simulink model "Pendulum6DOF"  (R2017a)
settings: Solver=ode45  StartTime=0.0  StopTime=500  MaxStep=0.01  RelTol=1e-3
settings Model: Creator=Charlie  LastModifiedBy=Charlie

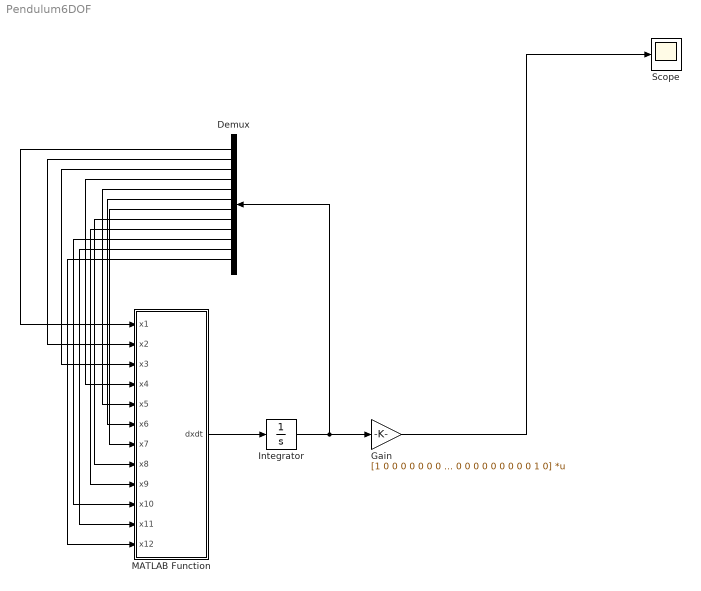
== system Pendulum6DOF ==
  Demux : Demux  Outputs=12
  Gain : Gain  Gain=[1 0 0 0 0 0 0 0 0 0 0 0; 0 0 1 0 0 0 0 0 0 0 0 0; 0 0 0 0 1 0 0 0 0 0 0 0; 0 0 0 0 0 0 1 0 0 0 0 0; 0 0 0 0 0 0 0 0 1 0 0 0; 0 0 0 0 0 0 0 0 0 0 1 0]  Multiplication=Matrix(K*u)
  Integrator : Integrator  InitialCondition=[pi-1;0;pi-0.2;0; 0;0; 1.5;0; 6;0; 0;0]
  MATLAB Function : MATLAB Function  TreatAsAtomicUnit=on
  Scope : Scope
  wires:
  Integrator/1 -> Demux/1, Gain/1
  Gain/1 -> Scope/1
  Demux/6 -> MATLAB Function/6(x6)
  Demux/5 -> MATLAB Function/5(x5)
  Demux/4 -> MATLAB Function/4(x4)
  Demux/3 -> MATLAB Function/3(x3)
  Demux/2 -> MATLAB Function/2(x2)
  Demux/1 -> MATLAB Function/1(x1)
  Demux/7 -> MATLAB Function/7(x7)
  Demux/8 -> MATLAB Function/8(x8)
  Demux/9 -> MATLAB Function/9(x9)
  Demux/10 -> MATLAB Function/10(x10)
  Demux/11 -> MATLAB Function/11(x11)
  Demux/12 -> MATLAB Function/12(x12)
  MATLAB Function/1(dxdt) -> Integrator/1

== matlab function Pendulum6DOF/MATLAB Function ==
  data: x1 input; dxdt output; x2 input; x3 input; x4 input; x5 input; x6 input; x7 input; x8 input; x9 input; x10 input; x11 input; x12 input
%function dxdt = dynamics(K,x)
function dxdt = dynamics(x1,x2,x3,x4,x5,x6,x7,x8,x9,x10,x11,x12)

dxdt = [x2;
    -((10430973*cos(x3)*sin(x1))/250000000 + (1029*x4^2*sin(2*x1))/5000000 + (50421*x4^2*cos(x1)^3*sin(x1))/50000 + (7066143*cos(x1)^2*cos(x3)*sin(x1))/250000 - (53851*x2*x4*sin(2*x3))/50000000 - (7066143*cos(x1)^2*cos(x3)^3*sin(x1))/250000000 + (10633*x2^2*cos(x1)*cos(x3)^2*sin(x1))/50000000 + (53851*x4^2*cos(x1)*cos(x3)^2*sin(x1))/50000000 - (31899*x6^2*cos(x1)*cos(x3)^2*sin(x1))/25000000 + (1029*x4*x6*cos(x1)^2*cos(x3))/1250000 + (50421*x4*x6*cos(x1)^4*cos(x3))/25000 + (7203*x2^2*cos(x1)^3*cos(x3)^2*sin(x1))/50000 - (7203*x2^2*cos(x1)^3*cos(x3)^4*sin(x1))/50000000 - (21609*x4^2*cos(x1)^3*cos(x3)^2*sin(x1))/25000000 - (7203*x4^2*cos(x1)^3*cos(x3)^4*sin(x1))/50000000 - (21609*x6^2*cos(x1)^3*cos(x3)^2*sin(x1))/25000 + (21609*x6^2*cos(x1)^3*cos(x3)^4*sin(x1))/25000000 + (21609*x4*x6*cos(x1)^2*cos(x3)^3)/12500000 - (3623109*x4*x6*cos(x1)^4*cos(x3)^3)/12500000 + (53851*x2*x4*cos(x1)^2*cos(x3)*sin(x3))/25000000 + (7203*x2*x4*cos(x1)^2*cos(x3)^3*sin(x3))/25000000 - (7203*x2*x4*cos(x1)^4*cos(x3)^3*sin(x3))/25000000 - (21609*x2*x6*cos(x1)*cos(x3)^2*sin(x1)*sin(x3))/12500000 + (7203*x2*x6*cos(x1)^3*cos(x3)^2*sin(x1)*sin(x3))/25000)/((50495431*cos(x1)^2)/50000000 + (53851*cos(x3)^2)/50000000 - (5386129*cos(x1)^2*cos(x3)^2)/2500000000 - (7203*cos(x1)^2*cos(x3)^4)/50000000 - (7210203*cos(x1)^4*cos(x3)^2)/50000000 + (7203*cos(x1)^4*cos(x3)^4)/25000000 + 1030519/2500000000);
    x4;
    ((50495431*x2*x4*sin(2*x1))/50000000 - (7076573973*cos(x1)*sin(x3))/250000000 + (7066143*cos(x1)^3*cos(x3)^2*sin(x3))/250000000 - (7213633*x2^2*cos(x1)^2*cos(x3)*sin(x3))/50000000 - (53851*x4^2*cos(x1)^2*cos(x3)*sin(x3))/50000000 - (3579891*x4^2*cos(x1)^4*cos(x3)*sin(x3))/25000000 + (21640899*x6^2*cos(x1)^2*cos(x3)*sin(x3))/25000000 + (21640899*x2*x6*cos(x1)^2*cos(x3))/12500000 + (7203*x2^2*cos(x1)^4*cos(x3)^3*sin(x3))/50000000 + (7203*x4^2*cos(x1)^4*cos(x3)^3*sin(x3))/50000000 - (21609*x6^2*cos(x1)^4*cos(x3)^3*sin(x3))/25000000 + (3579891*x2*x6*cos(x1)^2*cos(x3)^3)/12500000 - (7203*x2*x6*cos(x1)^4*cos(x3)^3)/25000 - (53851*x2*x4*cos(x1)*cos(x3)^2*sin(x1))/25000000 - (7210203*x2*x4*cos(x1)^3*cos(x3)^2*sin(x1))/25000000 + (7203*x2*x4*cos(x1)^3*cos(x3)^4*sin(x1))/25000000 + (3579891*x4*x6*cos(x1)^3*cos(x3)^2*sin(x1)*sin(x3))/12500000)/((50495431*cos(x1)^2)/50000000 + (53851*cos(x3)^2)/50000000 - (5386129*cos(x1)^2*cos(x3)^2)/2500000000 - (7203*cos(x1)^2*cos(x3)^4)/50000000 - (7210203*cos(x1)^4*cos(x3)^2)/50000000 + (7203*cos(x1)^4*cos(x3)^4)/25000000 + 1030519/2500000000);
    x6;
    -(147*((17157*x2*x4*cos(x3))/25000000 - (48069*cos(x3)*sin(x1)*sin(x3))/5000000 + (343*x4^2*cos(x1)^3*sin(x1)*sin(x3))/1000000 + (48069*cos(x1)^2*cos(x3)*sin(x1)*sin(x3))/5000000 - (17157*x2*x4*cos(x1)^2*cos(x3))/25000000 - (49*x2*x4*cos(x1)^2*cos(x3)^3)/500000 + (49*x2*x4*cos(x1)^4*cos(x3)^3)/500000 + (7*x4^2*cos(x1)*sin(x1)*sin(x3))/50000000 - (49*x2^2*cos(x1)*cos(x3)^2*sin(x1)*sin(x3))/1000000 + (147*x6^2*cos(x1)*cos(x3)^2*sin(x1)*sin(x3))/500000 + (14707*x2*x6*cos(x1)*cos(x3)^2*sin(x1))/25000000 + (49*x2*x6*cos(x1)*cos(x3)^4*sin(x1))/500000 + (7*x4*x6*cos(x1)^2*cos(x3)*sin(x3))/25000000 + (343*x4*x6*cos(x1)^4*cos(x3)*sin(x3))/500000 + (49*x2^2*cos(x1)^3*cos(x3)^2*sin(x1)*sin(x3))/1000000 - (49*x4^2*cos(x1)^3*cos(x3)^2*sin(x1)*sin(x3))/1000000 - (147*x6^2*cos(x1)^3*cos(x3)^2*sin(x1)*sin(x3))/500000 + (49*x2*x6*cos(x1)^3*cos(x3)^2*sin(x1))/500000 - (49*x2*x6*cos(x1)^3*cos(x3)^4*sin(x1))/250000 + (49*x4*x6*cos(x1)^2*cos(x3)^3*sin(x3))/500000 - (49*x4*x6*cos(x1)^4*cos(x3)^3*sin(x3))/250000))/(50*((50495431*cos(x1)^2)/50000000 + (53851*cos(x3)^2)/50000000 - (5386129*cos(x1)^2*cos(x3)^2)/2500000000 - (7203*cos(x1)^2*cos(x3)^4)/50000000 - (7210203*cos(x1)^4*cos(x3)^2)/50000000 + (7203*cos(x1)^4*cos(x3)^4)/25000000 + 1030519/2500000000));
    x8;
    ((1030519*x7*x12^2)/2500000000 - (1030519*x10*x12)/1250000000 - (50495431*x10*x12*cos(x1)^2)/25000000 - (53851*x10*x12*cos(x3)^2)/25000000 + (50495431*x7*x12^2*cos(x1)^2)/50000000 + (53851*x7*x12^2*cos(x3)^2)/50000000 - (5386129*x7*x12^2*cos(x1)^2*cos(x3)^2)/2500000000 - (7203*x7*x12^2*cos(x1)^2*cos(x3)^4)/50000000 - (7210203*x7*x12^2*cos(x1)^4*cos(x3)^2)/50000000 + (7203*x7*x12^2*cos(x1)^4*cos(x3)^4)/25000000 + (5386129*x10*x12*cos(x1)^2*cos(x3)^2)/1250000000 + (7203*x10*x12*cos(x1)^2*cos(x3)^4)/25000000 + (7210203*x10*x12*cos(x1)^4*cos(x3)^2)/25000000 - (7203*x10*x12*cos(x1)^4*cos(x3)^4)/12500000 - (336483*cos(x3)*cos(x5)*cos(x11)*sin(x3))/500000000 + (1030519*x2^2*cos(x5)*sin(x1)*sin(x11))/50000000000 - (1030519*x2^2*cos(x11)*sin(x1)*sin(x5))/50000000000 + (1030519*x6^2*cos(x5)*sin(x1)*sin(x11))/50000000000 - (1030519*x6^2*cos(x11)*sin(x1)*sin(x5))/50000000000 - (336483*cos(x3)*sin(x3)*sin(x5)*sin(x11))/500000000 + (1030519*x2*x6*cos(x1)*sin(x5)*sin(x11))/25000000000 + (50495431*x2^2*cos(x1)^3*cos(x5)*cos(x11)*sin(x3))/1000000000 + (2230529*x4^2*cos(x1)^3*cos(x5)*cos(x11)*sin(x3))/50000000000 + (50471421*x4^2*cos(x1)^5*cos(x5)*cos(x11)*sin(x3))/1000000000 + (50495431*x6^2*cos(x1)^3*cos(x5)*cos(x11)*sin(x3))/1000000000 + (336483*cos(x1)^2*cos(x3)*cos(x5)*cos(x11)*sin(x3))/250000000 + (7073209143*cos(x1)^4*cos(x3)*cos(x5)*cos(x11)*sin(x3))/5000000000 + (50495431*x2^2*cos(x1)^2*cos(x5)*sin(x1)*sin(x11))/1000000000 - (50495431*x2^2*cos(x1)^2*cos(x11)*sin(x1)*sin(x5))/1000000000 + (53851*x2^2*cos(x3)^2*cos(x5)*sin(x1)*sin(x11))/1000000000 - (53851*x2^2*cos(x3)^2*cos(x11)*sin(x1)*sin(x5))/1000000000 + (1030029*x4^2*cos(x1)^2*cos(x5)*sin(x1)*sin(x11))/50000000000 - (1030029*x4^2*cos(x1)^2*cos(x11)*sin(x1)*sin(x5))/50000000000 + (50471421*x4^2*cos(x1)^4*cos(x5)*sin(x1)*sin(x11))/1000000000 - (50471421*x4^2*cos(x1)^4*cos(x11)*sin(x1)*sin(x5))/1000000000 + (50495431*x6^2*cos(x1)^2*cos(x5)*sin(x1)*sin(x11))/1000000000 - (50495431*x6^2*cos(x1)^2*cos(x11)*sin(x1)*sin(x5))/1000000000 + (53851*x6^2*cos(x3)^2*cos(x5)*sin(x1)*sin(x11))/1000000000 - (53851*x6^2*cos(x3)^2*cos(x11)*sin(x1)*sin(x5))/1000000000 + (7066143*cos(x1)*cos(x3)^3*cos(x5)*sin(x1)*sin(x11))/5000000000 - (7066143*cos(x1)*cos(x3)^3*cos(x11)*sin(x1)*sin(x5))/5000000000 + (7073209143*cos(x1)^3*cos(x3)*cos(x5)*sin(x1)*sin(x11))/5000000000 - (7073209143*cos(x1)^3*cos(x3)*cos(x11)*sin(x1)*sin(x5))/5000000000 + (50495431*x2^2*cos(x1)^3*sin(x3)*sin(x5)*sin(x11))/1000000000 + (2230529*x4^2*cos(x1)^3*sin(x3)*sin(x5)*sin(x11))/50000000000 + (50471421*x4^2*cos(x1)^5*sin(x3)*sin(x5)*sin(x11))/1000000000 + (50495431*x6^2*cos(x1)^3*sin(x3)*sin(x5)*sin(x11))/1000000000 + (336483*cos(x1)^2*cos(x3)*sin(x3)*sin(x5)*sin(x11))/250000000 + (7073209143*cos(x1)^4*cos(x3)*sin(x3)*sin(x5)*sin(x11))/5000000000 + (50495431*x2*x6*cos(x1)^3*cos(x5)*cos(x11))/500000000 + (50495431*x2*x6*cos(x1)^3*sin(x5)*sin(x11))/500000000 + (7066143*cos(x1)^2*cos(x3)^3*cos(x5)*cos(x11)*sin(x3))/5000000000 - (7066143*cos(x1)^4*cos(x3)^3*cos(x5)*cos(x11)*sin(x3))/2500000000 - (7066143*cos(x1)^3*cos(x3)^3*cos(x5)*sin(x1)*sin(x11))/2500000000 + (7066143*cos(x1)^3*cos(x3)^3*cos(x11)*sin(x1)*sin(x5))/2500000000 + (7066143*cos(x1)^2*cos(x3)^3*sin(x3)*sin(x5)*sin(x11))/5000000000 - (7066143*cos(x1)^4*cos(x3)^3*sin(x3)*sin(x5)*sin(x11))/2500000000 + (1030519*x2^2*cos(x1)*cos(x5)*cos(x11)*sin(x3))/50000000000 + (49*x4^2*cos(x1)*cos(x5)*cos(x11)*sin(x3))/5000000000 + (1030519*x6^2*cos(x1)*cos(x5)*cos(x11)*sin(x3))/50000000000 + (336483*cos(x1)*cos(x3)*cos(x5)*sin(x1)*sin(x11))/500000000 - (336483*cos(x1)*cos(x3)*cos(x11)*sin(x1)*sin(x5))/500000000 + (1030519*x2^2*cos(x1)*sin(x3)*sin(x5)*sin(x11))/50000000000 + (49*x4^2*cos(x1)*sin(x3)*sin(x5)*sin(x11))/5000000000 + (1030519*x6^2*cos(x1)*sin(x3)*sin(x5)*sin(x11))/50000000000 + (1030519*x2*x6*cos(x1)*cos(x5)*cos(x11))/25000000000 + (50421*x2^2*cos(x1)*cos(x3)^2*sin(x3)*sin(x5)*sin(x11))/1000000000 + (74431*x6^2*cos(x1)*cos(x3)^2*sin(x3)*sin(x5)*sin(x11))/1000000000 + (2691521*x2*x6*cos(x1)*cos(x3)^2*cos(x5)*cos(x11))/25000000000 - (50421*x2*x6*cos(x1)*cos(x3)^4*cos(x5)*cos(x11))/500000000 - (53851*x4*x6*cos(x1)*cos(x3)^3*cos(x5)*sin(x11))/500000000 + (53851*x4*x6*cos(x1)*cos(x3)^3*cos(x11)*sin(x5))/500000000 - (2523741521*x4*x6*cos(x1)^3*cos(x3)*cos(x5)*sin(x11))/25000000000 + (2523741521*x4*x6*cos(x1)^3*cos(x3)*cos(x11)*sin(x5))/25000000000 + (50471421*x4*x6*cos(x1)^5*cos(x3)*cos(x5)*sin(x11))/500000000 - (50471421*x4*x6*cos(x1)^5*cos(x3)*cos(x11)*sin(x5))/500000000 + (2691521*x2*x6*cos(x1)*cos(x3)^2*sin(x5)*sin(x11))/25000000000 - (50421*x2*x6*cos(x1)*cos(x3)^4*sin(x5)*sin(x11))/500000000 - (5043129*x2^2*cos(x1)^3*cos(x3)^2*cos(x5)*cos(x11)*sin(x3))/50000000000 + (2520021*x4^2*cos(x1)^3*cos(x3)^2*cos(x5)*cos(x11)*sin(x3))/50000000000 - (50421*x4^2*cos(x1)^5*cos(x3)^2*cos(x5)*cos(x11)*sin(x3))/500000000 - (7444129*x6^2*cos(x1)^3*cos(x3)^2*cos(x5)*cos(x11)*sin(x3))/50000000000 - (50421*x6^2*cos(x1)^3*cos(x3)^4*cos(x5)*cos(x11)*sin(x3))/1000000000 - (50471421*x6^2*cos(x1)^5*cos(x3)^2*cos(x5)*cos(x11)*sin(x3))/1000000000 + (50421*x6^2*cos(x1)^5*cos(x3)^4*cos(x5)*cos(x11)*sin(x3))/500000000 - (5214629*x2^2*cos(x1)^2*cos(x3)^2*cos(x5)*sin(x1)*sin(x11))/50000000000 + (5214629*x2^2*cos(x1)^2*cos(x3)^2*cos(x11)*sin(x1)*sin(x5))/50000000000 + (2691521*x4^2*cos(x1)^2*cos(x3)^2*cos(x5)*sin(x1)*sin(x11))/50000000000 - (2691521*x4^2*cos(x1)^2*cos(x3)^2*cos(x11)*sin(x1)*sin(x5))/50000000000 - (50421*x4^2*cos(x1)^4*cos(x3)^2*cos(x5)*sin(x1)*sin(x11))/500000000 + (50421*x4^2*cos(x1)^4*cos(x3)^2*cos(x11)*sin(x1)*sin(x5))/500000000 - (6415129*x6^2*cos(x1)^2*cos(x3)^2*cos(x5)*sin(x1)*sin(x11))/50000000000 + (6415129*x6^2*cos(x1)^2*cos(x3)^2*cos(x11)*sin(x1)*sin(x5))/50000000000 - (50421*x6^2*cos(x1)^2*cos(x3)^4*cos(x5)*sin(x1)*sin(x11))/1000000000 + (50421*x6^2*cos(x1)^2*cos(x3)^4*cos(x11)*sin(x1)*sin(x5))/1000000000 - (50471421*x6^2*cos(x1)^4*cos(x3)^2*cos(x5)*sin(x1)*sin(x11))/1000000000 + (50471421*x6^2*cos(x1)^4*cos(x3)^2*cos(x11)*sin(x1)*sin(x5))/1000000000 + (50421*x6^2*cos(x1)^4*cos(x3)^4*cos(x5)*sin(x1)*sin(x11))/500000000 - (50421*x6^2*cos(x1)^4*cos(x3)^4*cos(x11)*sin(x1)*sin(x5))/500000000 - (5043129*x2^2*cos(x1)^3*cos(x3)^2*sin(x3)*sin(x5)*sin(x11))/50000000000 + (2520021*x4^2*cos(x1)^3*cos(x3)^2*sin(x3)*sin(x5)*sin(x11))/50000000000 - (50421*x4^2*cos(x1)^5*cos(x3)^2*sin(x3)*sin(x5)*sin(x11))/500000000 - (7444129*x6^2*cos(x1)^3*cos(x3)^2*sin(x3)*sin(x5)*sin(x11))/50000000000 - (50421*x6^2*cos(x1)^3*cos(x3)^4*sin(x3)*sin(x5)*sin(x11))/1000000000 - (50471421*x6^2*cos(x1)^5*cos(x3)^2*sin(x3)*sin(x5)*sin(x11))/1000000000 + (50421*x6^2*cos(x1)^5*cos(x3)^4*sin(x3)*sin(x5)*sin(x11))/500000000 - (50599703*x2*x6*cos(x1)^3*cos(x3)^2*cos(x5)*cos(x11))/500000000 + (50421*x2*x6*cos(x1)^3*cos(x3)^4*cos(x5)*cos(x11))/250000000 + (158123*x4*x6*cos(x1)^3*cos(x3)^3*cos(x5)*sin(x11))/500000000 - (158123*x4*x6*cos(x1)^3*cos(x3)^3*cos(x11)*sin(x5))/500000000 - (50421*x4*x6*cos(x1)^5*cos(x3)^3*cos(x5)*sin(x11))/250000000 + (50421*x4*x6*cos(x1)^5*cos(x3)^3*cos(x11)*sin(x5))/250000000 - (50599703*x2*x6*cos(x1)^3*cos(x3)^2*sin(x5)*sin(x11))/500000000 + (50421*x2*x6*cos(x1)^3*cos(x3)^4*sin(x5)*sin(x11))/250000000 + (120099*x2*x4*cos(x3)*cos(x5)*cos(x11)*sin(x1))/2500000000 - (1030519*x4*x6*cos(x1)*cos(x3)*cos(x5)*sin(x11))/25000000000 + (1030519*x4*x6*cos(x1)*cos(x3)*cos(x11)*sin(x5))/25000000000 + (120099*x2*x4*cos(x3)*sin(x1)*sin(x5)*sin(x11))/2500000000 + (1030519*x2*x6*cos(x5)*sin(x1)*sin(x3)*sin(x11))/25000000000 - (1030519*x2*x6*cos(x11)*sin(x1)*sin(x3)*sin(x5))/25000000000 + (50421*x2^2*cos(x1)*cos(x3)^2*cos(x5)*cos(x11)*sin(x3))/1000000000 + (74431*x6^2*cos(x1)*cos(x3)^2*cos(x5)*cos(x11)*sin(x3))/1000000000 - (170471*x2*x4*cos(x1)^2*cos(x3)*cos(x5)*cos(x11)*sin(x1))/25000000000 + (170471*x2*x4*cos(x1)^3*cos(x3)*cos(x5)*sin(x3)*sin(x11))/25000000000 - (170471*x2*x4*cos(x1)^3*cos(x3)*cos(x11)*sin(x3)*sin(x5))/25000000000 - (170471*x2*x4*cos(x1)^2*cos(x3)*sin(x1)*sin(x5)*sin(x11))/25000000000 + (50495431*x2*x6*cos(x1)^2*cos(x5)*sin(x1)*sin(x3)*sin(x11))/500000000 - (50495431*x2*x6*cos(x1)^2*cos(x11)*sin(x1)*sin(x3)*sin(x5))/500000000 + (53851*x2*x6*cos(x3)^2*cos(x5)*sin(x1)*sin(x3)*sin(x11))/500000000 - (53851*x2*x6*cos(x3)^2*cos(x11)*sin(x1)*sin(x3)*sin(x5))/500000000 - (1029*x2*x4*cos(x1)^2*cos(x3)^3*cos(x5)*cos(x11)*sin(x1))/25000000000 - (1029*x2*x4*cos(x1)^2*cos(x3)^3*sin(x1)*sin(x5)*sin(x11))/25000000000 - (170471*x2*x4*cos(x1)*cos(x3)*cos(x5)*sin(x3)*sin(x11))/25000000000 + (170471*x2*x4*cos(x1)*cos(x3)*cos(x11)*sin(x3)*sin(x5))/25000000000 - (1030029*x4*x6*cos(x1)^2*cos(x3)*sin(x1)*sin(x3)*sin(x5)*sin(x11))/25000000000 - (50471421*x4*x6*cos(x1)^4*cos(x3)*sin(x1)*sin(x3)*sin(x5)*sin(x11))/500000000 - (50421*x4*x6*cos(x1)^2*cos(x3)^3*cos(x5)*cos(x11)*sin(x1)*sin(x3))/500000000 + (50421*x4*x6*cos(x1)^4*cos(x3)^3*cos(x5)*cos(x11)*sin(x1)*sin(x3))/250000000 - (53851*x2*x6*cos(x1)^2*cos(x3)^2*cos(x5)*sin(x1)*sin(x3)*sin(x11))/250000000 + (53851*x2*x6*cos(x1)^2*cos(x3)^2*cos(x11)*sin(x1)*sin(x3)*sin(x5))/250000000 - (50421*x4*x6*cos(x1)^2*cos(x3)^3*sin(x1)*sin(x3)*sin(x5)*sin(x11))/500000000 + (50421*x4*x6*cos(x1)^4*cos(x3)^3*sin(x1)*sin(x3)*sin(x5)*sin(x11))/250000000 - (1030029*x4*x6*cos(x1)^2*cos(x3)*cos(x5)*cos(x11)*sin(x1)*sin(x3))/25000000000 - (50471421*x4*x6*cos(x1)^4*cos(x3)*cos(x5)*cos(x11)*sin(x1)*sin(x3))/500000000)/((50495431*cos(x1)^2)/50000000 + (53851*cos(x3)^2)/50000000 - (5386129*cos(x1)^2*cos(x3)^2)/2500000000 - (7203*cos(x1)^2*cos(x3)^4)/50000000 - (7210203*cos(x1)^4*cos(x3)^2)/50000000 + (7203*cos(x1)^4*cos(x3)^4)/25000000 + 1030519/2500000000);
    x10;
    -((5386129*x9*x12^2*cos(x1)^2*cos(x3)^2)/2500000000 - (1030519*x9*x12^2)/2500000000 - (50495431*x8*x12*cos(x1)^2)/25000000 - (53851*x8*x12*cos(x3)^2)/25000000 - (50495431*x9*x12^2*cos(x1)^2)/50000000 - (53851*x9*x12^2*cos(x3)^2)/50000000 - (1030519*x8*x12)/1250000000 + (7203*x9*x12^2*cos(x1)^2*cos(x3)^4)/50000000 + (7210203*x9*x12^2*cos(x1)^4*cos(x3)^2)/50000000 - (7203*x9*x12^2*cos(x1)^4*cos(x3)^4)/25000000 + (5386129*x8*x12*cos(x1)^2*cos(x3)^2)/1250000000 + (7203*x8*x12*cos(x1)^2*cos(x3)^4)/25000000 + (7210203*x8*x12*cos(x1)^4*cos(x3)^2)/25000000 - (7203*x8*x12*cos(x1)^4*cos(x3)^4)/12500000 + (1030519*x2^2*cos(x5)*cos(x11)*sin(x1))/50000000000 + (1030519*x6^2*cos(x5)*cos(x11)*sin(x1))/50000000000 + (336483*cos(x3)*cos(x5)*sin(x3)*sin(x11))/500000000 - (336483*cos(x3)*cos(x11)*sin(x3)*sin(x5))/500000000 + (1030519*x2^2*sin(x1)*sin(x5)*sin(x11))/50000000000 + (1030519*x6^2*sin(x1)*sin(x5)*sin(x11))/50000000000 + (50495431*x2^2*cos(x1)^2*cos(x5)*cos(x11)*sin(x1))/1000000000 + (53851*x2^2*cos(x3)^2*cos(x5)*cos(x11)*sin(x1))/1000000000 + (1030029*x4^2*cos(x1)^2*cos(x5)*cos(x11)*sin(x1))/50000000000 + (50471421*x4^2*cos(x1)^4*cos(x5)*cos(x11)*sin(x1))/1000000000 + (50495431*x6^2*cos(x1)^2*cos(x5)*cos(x11)*sin(x1))/1000000000 + (53851*x6^2*cos(x3)^2*cos(x5)*cos(x11)*sin(x1))/1000000000 + (7066143*cos(x1)*cos(x3)^3*cos(x5)*cos(x11)*sin(x1))/5000000000 + (7073209143*cos(x1)^3*cos(x3)*cos(x5)*cos(x11)*sin(x1))/5000000000 - (50495431*x2^2*cos(x1)^3*cos(x5)*sin(x3)*sin(x11))/1000000000 + (50495431*x2^2*cos(x1)^3*cos(x11)*sin(x3)*sin(x5))/1000000000 - (2230529*x4^2*cos(x1)^3*cos(x5)*sin(x3)*sin(x11))/50000000000 + (2230529*x4^2*cos(x1)^3*cos(x11)*sin(x3)*sin(x5))/50000000000 - (50471421*x4^2*cos(x1)^5*cos(x5)*sin(x3)*sin(x11))/1000000000 + (50471421*x4^2*cos(x1)^5*cos(x11)*sin(x3)*sin(x5))/1000000000 - (50495431*x6^2*cos(x1)^3*cos(x5)*sin(x3)*sin(x11))/1000000000 + (50495431*x6^2*cos(x1)^3*cos(x11)*sin(x3)*sin(x5))/1000000000 - (336483*cos(x1)^2*cos(x3)*cos(x5)*sin(x3)*sin(x11))/250000000 + (336483*cos(x1)^2*cos(x3)*cos(x11)*sin(x3)*sin(x5))/250000000 - (7073209143*cos(x1)^4*cos(x3)*cos(x5)*sin(x3)*sin(x11))/5000000000 + (7073209143*cos(x1)^4*cos(x3)*cos(x11)*sin(x3)*sin(x5))/5000000000 + (50495431*x2^2*cos(x1)^2*sin(x1)*sin(x5)*sin(x11))/1000000000 + (53851*x2^2*cos(x3)^2*sin(x1)*sin(x5)*sin(x11))/1000000000 + (1030029*x4^2*cos(x1)^2*sin(x1)*sin(x5)*sin(x11))/50000000000 + (50471421*x4^2*cos(x1)^4*sin(x1)*sin(x5)*sin(x11))/1000000000 + (50495431*x6^2*cos(x1)^2*sin(x1)*sin(x5)*sin(x11))/1000000000 + (53851*x6^2*cos(x3)^2*sin(x1)*sin(x5)*sin(x11))/1000000000 + (7066143*cos(x1)*cos(x3)^3*sin(x1)*sin(x5)*sin(x11))/5000000000 + (7073209143*cos(x1)^3*cos(x3)*sin(x1)*sin(x5)*sin(x11))/5000000000 - (50495431*x2*x6*cos(x1)^3*cos(x5)*sin(x11))/500000000 + (50495431*x2*x6*cos(x1)^3*cos(x11)*sin(x5))/500000000 - (7066143*cos(x1)^3*cos(x3)^3*cos(x5)*cos(x11)*sin(x1))/2500000000 - (7066143*cos(x1)^2*cos(x3)^3*cos(x5)*sin(x3)*sin(x11))/5000000000 + (7066143*cos(x1)^2*cos(x3)^3*cos(x11)*sin(x3)*sin(x5))/5000000000 + (7066143*cos(x1)^4*cos(x3)^3*cos(x5)*sin(x3)*sin(x11))/2500000000 - (7066143*cos(x1)^4*cos(x3)^3*cos(x11)*sin(x3)*sin(x5))/2500000000 - (7066143*cos(x1)^3*cos(x3)^3*sin(x1)*sin(x5)*sin(x11))/2500000000 + (336483*cos(x1)*cos(x3)*cos(x5)*cos(x11)*sin(x1))/500000000 - (1030519*x2^2*cos(x1)*cos(x5)*sin(x3)*sin(x11))/50000000000 + (1030519*x2^2*cos(x1)*cos(x11)*sin(x3)*sin(x5))/50000000000 - (49*x4^2*cos(x1)*cos(x5)*sin(x3)*sin(x11))/5000000000 + (49*x4^2*cos(x1)*cos(x11)*sin(x3)*sin(x5))/5000000000 - (1030519*x6^2*cos(x1)*cos(x5)*sin(x3)*sin(x11))/50000000000 + (1030519*x6^2*cos(x1)*cos(x11)*sin(x3)*sin(x5))/50000000000 + (336483*cos(x1)*cos(x3)*sin(x1)*sin(x5)*sin(x11))/500000000 - (1030519*x2*x6*cos(x1)*cos(x5)*sin(x11))/25000000000 + (1030519*x2*x6*cos(x1)*cos(x11)*sin(x5))/25000000000 - (53851*x4*x6*cos(x1)*cos(x3)^3*cos(x5)*cos(x11))/500000000 - (2523741521*x4*x6*cos(x1)^3*cos(x3)*cos(x5)*cos(x11))/25000000000 + (50471421*x4*x6*cos(x1)^5*cos(x3)*cos(x5)*cos(x11))/500000000 - (2691521*x2*x6*cos(x1)*cos(x3)^2*cos(x5)*sin(x11))/25000000000 + (2691521*x2*x6*cos(x1)*cos(x3)^2*cos(x11)*sin(x5))/25000000000 + (50421*x2*x6*cos(x1)*cos(x3)^4*cos(x5)*sin(x11))/500000000 - (50421*x2*x6*cos(x1)*cos(x3)^4*cos(x11)*sin(x5))/500000000 - (53851*x4*x6*cos(x1)*cos(x3)^3*sin(x5)*sin(x11))/500000000 - (2523741521*x4*x6*cos(x1)^3*cos(x3)*sin(x5)*sin(x11))/25000000000 + (50471421*x4*x6*cos(x1)^5*cos(x3)*sin(x5)*sin(x11))/500000000 - (5214629*x2^2*cos(x1)^2*cos(x3)^2*cos(x5)*cos(x11)*sin(x1))/50000000000 + (2691521*x4^2*cos(x1)^2*cos(x3)^2*cos(x5)*cos(x11)*sin(x1))/50000000000 - (50421*x4^2*cos(x1)^4*cos(x3)^2*cos(x5)*cos(x11)*sin(x1))/500000000 - (6415129*x6^2*cos(x1)^2*cos(x3)^2*cos(x5)*cos(x11)*sin(x1))/50000000000 - (50421*x6^2*cos(x1)^2*cos(x3)^4*cos(x5)*cos(x11)*sin(x1))/1000000000 - (50471421*x6^2*cos(x1)^4*cos(x3)^2*cos(x5)*cos(x11)*sin(x1))/1000000000 + (50421*x6^2*cos(x1)^4*cos(x3)^4*cos(x5)*cos(x11)*sin(x1))/500000000 + (5043129*x2^2*cos(x1)^3*cos(x3)^2*cos(x5)*sin(x3)*sin(x11))/50000000000 - (5043129*x2^2*cos(x1)^3*cos(x3)^2*cos(x11)*sin(x3)*sin(x5))/50000000000 - (2520021*x4^2*cos(x1)^3*cos(x3)^2*cos(x5)*sin(x3)*sin(x11))/50000000000 + (2520021*x4^2*cos(x1)^3*cos(x3)^2*cos(x11)*sin(x3)*sin(x5))/50000000000 + (50421*x4^2*cos(x1)^5*cos(x3)^2*cos(x5)*sin(x3)*sin(x11))/500000000 - (50421*x4^2*cos(x1)^5*cos(x3)^2*cos(x11)*sin(x3)*sin(x5))/500000000 + (7444129*x6^2*cos(x1)^3*cos(x3)^2*cos(x5)*sin(x3)*sin(x11))/50000000000 - (7444129*x6^2*cos(x1)^3*cos(x3)^2*cos(x11)*sin(x3)*sin(x5))/50000000000 + (50421*x6^2*cos(x1)^3*cos(x3)^4*cos(x5)*sin(x3)*sin(x11))/1000000000 - (50421*x6^2*cos(x1)^3*cos(x3)^4*cos(x11)*sin(x3)*sin(x5))/1000000000 + (50471421*x6^2*cos(x1)^5*cos(x3)^2*cos(x5)*sin(x3)*sin(x11))/1000000000 - (50471421*x6^2*cos(x1)^5*cos(x3)^2*cos(x11)*sin(x3)*sin(x5))/1000000000 - (50421*x6^2*cos(x1)^5*cos(x3)^4*cos(x5)*sin(x3)*sin(x11))/500000000 + (50421*x6^2*cos(x1)^5*cos(x3)^4*cos(x11)*sin(x3)*sin(x5))/500000000 - (5214629*x2^2*cos(x1)^2*cos(x3)^2*sin(x1)*sin(x5)*sin(x11))/50000000000 + (2691521*x4^2*cos(x1)^2*cos(x3)^2*sin(x1)*sin(x5)*sin(x11))/50000000000 - (50421*x4^2*cos(x1)^4*cos(x3)^2*sin(x1)*sin(x5)*sin(x11))/500000000 - (6415129*x6^2*cos(x1)^2*cos(x3)^2*sin(x1)*sin(x5)*sin(x11))/50000000000 - (50421*x6^2*cos(x1)^2*cos(x3)^4*sin(x1)*sin(x5)*sin(x11))/1000000000 - (50471421*x6^2*cos(x1)^4*cos(x3)^2*sin(x1)*sin(x5)*sin(x11))/1000000000 + (50421*x6^2*cos(x1)^4*cos(x3)^4*sin(x1)*sin(x5)*sin(x11))/500000000 + (158123*x4*x6*cos(x1)^3*cos(x3)^3*cos(x5)*cos(x11))/500000000 - (50421*x4*x6*cos(x1)^5*cos(x3)^3*cos(x5)*cos(x11))/250000000 + (50599703*x2*x6*cos(x1)^3*cos(x3)^2*cos(x5)*sin(x11))/500000000 - (50599703*x2*x6*cos(x1)^3*cos(x3)^2*cos(x11)*sin(x5))/500000000 - (50421*x2*x6*cos(x1)^3*cos(x3)^4*cos(x5)*sin(x11))/250000000 + (50421*x2*x6*cos(x1)^3*cos(x3)^4*cos(x11)*sin(x5))/250000000 + (158123*x4*x6*cos(x1)^3*cos(x3)^3*sin(x5)*sin(x11))/500000000 - (50421*x4*x6*cos(x1)^5*cos(x3)^3*sin(x5)*sin(x11))/250000000 - (1030519*x4*x6*cos(x1)*cos(x3)*cos(x5)*cos(x11))/25000000000 - (120099*x2*x4*cos(x3)*cos(x5)*sin(x1)*sin(x11))/2500000000 + (120099*x2*x4*cos(x3)*cos(x11)*sin(x1)*sin(x5))/2500000000 + (1030519*x2*x6*cos(x5)*cos(x11)*sin(x1)*sin(x3))/25000000000 - (1030519*x4*x6*cos(x1)*cos(x3)*sin(x5)*sin(x11))/25000000000 + (1030519*x2*x6*sin(x1)*sin(x3)*sin(x5)*sin(x11))/25000000000 - (50421*x2^2*cos(x1)*cos(x3)^2*cos(x5)*sin(x3)*sin(x11))/1000000000 + (50421*x2^2*cos(x1)*cos(x3)^2*cos(x11)*sin(x3)*sin(x5))/1000000000 - (74431*x6^2*cos(x1)*cos(x3)^2*cos(x5)*sin(x3)*sin(x11))/1000000000 + (74431*x6^2*cos(x1)*cos(x3)^2*cos(x11)*sin(x3)*sin(x5))/1000000000 + (170471*x2*x4*cos(x1)^3*cos(x3)*cos(x5)*cos(x11)*sin(x3))/25000000000 + (170471*x2*x4*cos(x1)^2*cos(x3)*cos(x5)*sin(x1)*sin(x11))/25000000000 - (170471*x2*x4*cos(x1)^2*cos(x3)*cos(x11)*sin(x1)*sin(x5))/25000000000 + (50495431*x2*x6*cos(x1)^2*cos(x5)*cos(x11)*sin(x1)*sin(x3))/500000000 + (53851*x2*x6*cos(x3)^2*cos(x5)*cos(x11)*sin(x1)*sin(x3))/500000000 + (170471*x2*x4*cos(x1)^3*cos(x3)*sin(x3)*sin(x5)*sin(x11))/25000000000 + (50495431*x2*x6*cos(x1)^2*sin(x1)*sin(x3)*sin(x5)*sin(x11))/500000000 + (53851*x2*x6*cos(x3)^2*sin(x1)*sin(x3)*sin(x5)*sin(x11))/500000000 + (1029*x2*x4*cos(x1)^2*cos(x3)^3*cos(x5)*sin(x1)*sin(x11))/25000000000 - (1029*x2*x4*cos(x1)^2*cos(x3)^3*cos(x11)*sin(x1)*sin(x5))/25000000000 - (170471*x2*x4*cos(x1)*cos(x3)*cos(x5)*cos(x11)*sin(x3))/25000000000 - (170471*x2*x4*cos(x1)*cos(x3)*sin(x3)*sin(x5)*sin(x11))/25000000000 + (1030029*x4*x6*cos(x1)^2*cos(x3)*cos(x5)*sin(x1)*sin(x3)*sin(x11))/25000000000 - (1030029*x4*x6*cos(x1)^2*cos(x3)*cos(x11)*sin(x1)*sin(x3)*sin(x5))/25000000000 + (50471421*x4*x6*cos(x1)^4*cos(x3)*cos(x5)*sin(x1)*sin(x3)*sin(x11))/500000000 - (50471421*x4*x6*cos(x1)^4*cos(x3)*cos(x11)*sin(x1)*sin(x3)*sin(x5))/500000000 - (53851*x2*x6*cos(x1)^2*cos(x3)^2*cos(x5)*cos(x11)*sin(x1)*sin(x3))/250000000 + (50421*x4*x6*cos(x1)^2*cos(x3)^3*cos(x5)*sin(x1)*sin(x3)*sin(x11))/500000000 - (50421*x4*x6*cos(x1)^2*cos(x3)^3*cos(x11)*sin(x1)*sin(x3)*sin(x5))/500000000 - (50421*x4*x6*cos(x1)^4*cos(x3)^3*cos(x5)*sin(x1)*sin(x3)*sin(x11))/250000000 + (50421*x4*x6*cos(x1)^4*cos(x3)^3*cos(x11)*sin(x1)*sin(x3)*sin(x5))/250000000 - (53851*x2*x6*cos(x1)^2*cos(x3)^2*sin(x1)*sin(x3)*sin(x5)*sin(x11))/250000000)/((50495431*cos(x1)^2)/50000000 + (53851*cos(x3)^2)/50000000 - (5386129*cos(x1)^2*cos(x3)^2)/2500000000 - (7203*cos(x1)^2*cos(x3)^4)/50000000 - (7210203*cos(x1)^4*cos(x3)^2)/50000000 + (7203*cos(x1)^4*cos(x3)^4)/25000000 + 1030519/2500000000);
    x12;
    0]

end
